simulink model "dk_hoi_tiep_tuyen_tinh_hoa_r2015a"  (R2015a)
settings: Solver=ode4  SolverMode=SingleTasking  StartTime=0.0  StopTime=30  FixedStep=0.001  RelTol=1e-3
settings Model: CovMetricSettings=dwe  CovHtmlReporting=off  covSaveCumulativeToWorkspaceVar=off  CovSaveSingleToWorkspaceVar=off  CovExternalEMLEnable=on  Creator=ryell  LastModifiedBy=ryell
settings DataIOCC: LimitDataPoints=off  SaveFormat=Dataset
settings DebuggingCC: SFUnexpectedBacktrackingDiag=error  SFNoUnconditionalDefaultTransitionDiag=error
settings HardwareCC: ProdBitPerPointer=64  ProdLargestAtomicFloat=Float  ProdIntDivRoundTo=Zero  ProdEndianess=LittleEndian  ProdHWDeviceType=Specified
settings ModelReferenceCC: PropagateSignalLabelsOutOfModel=on
settings GRTTargetCC: TargetLangStandard=C99 (ISO)  GeneratePreprocessorConditionals=Use local settings

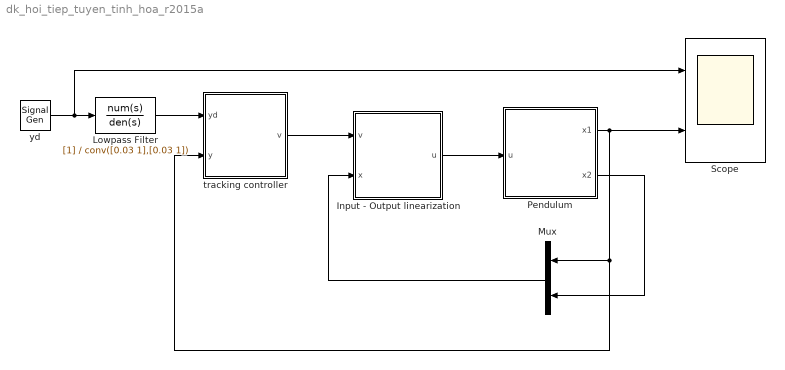
== system dk_hoi_tiep_tuyen_tinh_hoa_r2015a ==
  Input - Output linearization : Subsystem  mask{g=9.81, l=0.2, m=0.5, B=0.05}
  Lowpass Filter : TransferFcn  Denominator=conv([0.03 1],[0.03 1])
  Mux : Mux  Inputs=2
  Pendulum : Subsystem  mask{g=9.81, l=0.2, m=0.5, B=0.05, x1_init=0, x2_init=0}
      mask prompts: g "Gia toc trong truong"; l "Chieu dai thanh treo"; m "Khoi luong vat nang"; B "He so ma sat"; x1_init "Gia tri goc ban dau"; x2_init "Gia tri van toc goc ban dau"
  Scope : Scope  NumInputPorts=2
      settings: TimeRange=auto  MaxDataPoints=5000  SaveToWorkspace=off  SaveName=ScopeData  YMin=-0.6545~-5  YMax=0.6545~5  SampleTime=-1
  tracking controller : Subsystem
  yd : SignalGenerator  WaveForm=square  Amplitude=pi/6  Frequency=0.1
  wires:
  Input - Output linearization/1(u) -> Pendulum/1(u)
  Pendulum/2(x2) -> Mux/2
  Pendulum/1(x1) -> Scope/2, tracking controller/2(y), Mux/1
  Mux/1 -> Input - Output linearization/2(x)
  tracking controller/1(v) -> Input - Output linearization/1(v)
  yd/1 -> Scope/1, Lowpass Filter/1
  Lowpass Filter/1 -> tracking controller/1(yd)

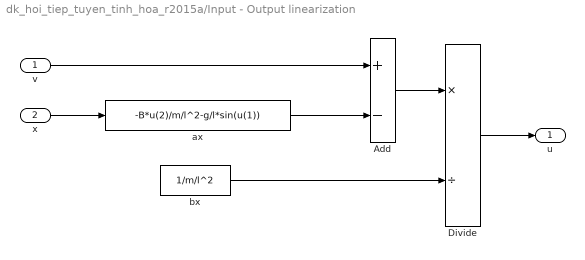
== system dk_hoi_tiep_tuyen_tinh_hoa_r2015a/Input - Output linearization ==
  v : Inport
  x : Inport  Port=2
  Add : Sum  Inputs=+-
  Divide : Product  Inputs=*/
  ax : Fcn  Expr=-B*u(2)/m/l^2-g/l*sin(u(1))
  bx : Constant  Value=1/m/l^2
  u : Outport
  wires:
  v/1 -> Add/1
  x/1 -> ax/1
  ax/1 -> Add/2
  Add/1 -> Divide/1
  bx/1 -> Divide/2
  Divide/1 -> u/1

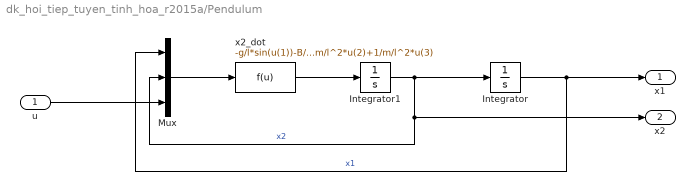
== system dk_hoi_tiep_tuyen_tinh_hoa_r2015a/Pendulum ==
  u : Inport
  Integrator : Integrator  InitialCondition=x1_init
  Integrator1 : Integrator  InitialCondition=x2_init
  Mux : Mux  Inputs=3
  x2_dot : Fcn  Expr=-g/l*sin(u(1))-B/m/l^2*u(2)+1/m/l^2*u(3)
  x1 : Outport
  x2 : Outport  Port=2
  wires:
  Integrator1/1 -> x2/1, Mux/2, Integrator/1  "x2"
  u/1 -> Mux/3
  x2_dot/1 -> Integrator1/1
  Integrator/1 -> x1/1, Mux/1  "x1"
  Mux/1 -> x2_dot/1

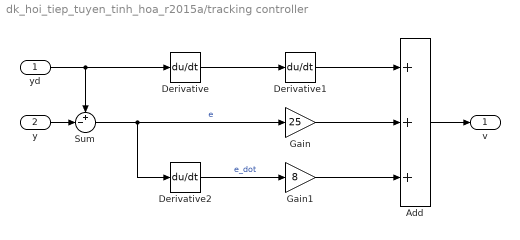
== system dk_hoi_tiep_tuyen_tinh_hoa_r2015a/tracking controller ==
  yd : Inport
  y : Inport  Port=2
  Add : Sum  Inputs=3
  Derivative : Derivative
  Derivative1 : Derivative
  Derivative2 : Derivative
  Gain : Gain  Gain=25
  Gain1 : Gain  Gain=8
  Sum : Sum  Inputs=+-|
  v : Outport
  wires:
  y/1 -> Sum/2
  yd/1 -> Derivative/1, Sum/1
  Derivative/1 -> Derivative1/1
  Gain/1 -> Add/2
  Gain1/1 -> Add/3
  Derivative1/1 -> Add/1
  Derivative2/1 -> Gain1/1  "e_dot"
  Sum/1 -> Derivative2/1, Gain/1  "e"
  Add/1 -> v/1
